simulink model "active_pendulum"  (R2020b)
settings: Solver=VariableStepAuto  StartTime=0.0  StopTime=2  RelTol=1e-3
values from neighbouring files (symbols this model uses):
  CONTROLLER_SAT = 5    [constants.m]
  DRIVER_SAT = 16    [constants.m]
  SENSOR_GAIN = 1024 / 2*pi    (= 1608.49543864)    [constants.m]
settings Model: Creator=matti  LastModifiedBy=matti

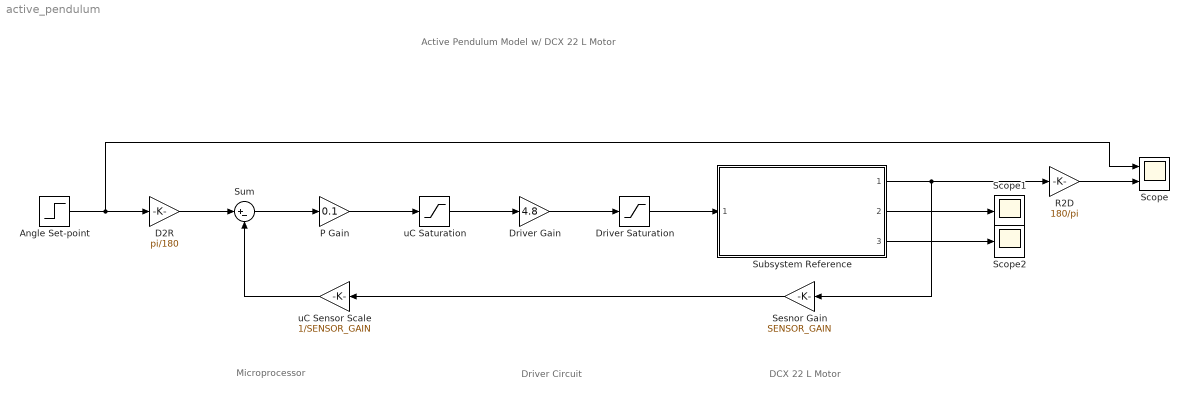
== system active_pendulum ==
  note: DCX 22 L Motor
  note: Driver Circuit
  note: Microprocessor
  note: Active Pendulum Model w/ DCX 22 L Motor
  Angle Set-point : Step  Time=0.1  After=45  SampleTime=0
  D2R : Gain  Gain=pi/180
  Driver Gain : Gain  Gain=4.8
  Driver Saturation : Saturate  UpperLimit=DRIVER_SAT  LowerLimit=-DRIVER_SAT
  P Gain : Gain  Gain=0.1
  R2D : Gain  Gain=180/pi
  Scope : Scope  NumInputPorts=2
  Scope1 : Scope
  Scope2 : Scope
  Sesnor Gain : Gain  Gain=SENSOR_GAIN
  Subsystem Reference : Subsystem  ReferencedSubsystem=dcx_22l
  Sum : Sum  Inputs=|+-
  uC Saturation : Saturate  UpperLimit=CONTROLLER_SAT  LowerLimit=-CONTROLLER_SAT
  uC Sensor Scale : Gain  Gain=1/SENSOR_GAIN
  wires:
  Sum/1 -> P Gain/1
  D2R/1 -> Sum/1
  Angle Set-point/1 -> Scope/1, D2R/1
  Subsystem Reference/1 -> Sesnor Gain/1, R2D/1
  R2D/1 -> Scope/2
  Subsystem Reference/2 -> Scope1/1
  Driver Saturation/1 -> Subsystem Reference/1
  Driver Gain/1 -> Driver Saturation/1
  P Gain/1 -> uC Saturation/1
  uC Saturation/1 -> Driver Gain/1
  Subsystem Reference/3 -> Scope2/1
  Sesnor Gain/1 -> uC Sensor Scale/1
  uC Sensor Scale/1 -> Sum/2
